simulink model "design_lqr_v1"  (R2019b)
settings: Solver=VariableStepAuto  StartTime=0.0  StopTime=10  RelTol=1e-3
values from neighbouring files (symbols this model uses):
  Ac = [A-B*F B*F;zeros(1*9) A-Ke*C1]    [design_hinfinity.m]    (also in design_lqr_m.m = [A-B*F B*F;zeros(9) A-Ke*C1]; design_v1.m)
  Bc = 1.0e+03*[ ... (first row only)    [design_hinfinity.m]    (also in design_lqr_m.m = [B*G;Zero_tem]; design_v1.m)
  Cc = [ 1     0     0     0     0     0     0     0     0  0     0     0     0     0     0     0     0     0 ... (first row only)    [design_hinfinity.m]    (also in design_lqr_m.m = [C1 zeros(9)]; design_v1.m)
  Rref = [0;0;0]    [design_lqr_m.m]    (also in design_v1.m)
  Vw = [ ... (first row only)    [design_hinfinity.m]    (also in design_lqr_m.m = [E;E]; design_v1.m = [E;E-Ke*[0;0;1;1;0;0;1;0;0]])
  x0 = [0 0 0 0 0 0 0 0 0;0 -0.1 0 0 0 0 0 0 0;0 0 0 0 0 0 0 0 0;0 0 0 0 0 0 0 0 0;0 0 0 0 0 0 0 0 0;0 0 0 0 0 0 0 0 0;0 0 0 0 0 0 0 0 0;0 0 0 0 0 0 0 0 0;0 0 0 0 0 0 0 0  0.1;0 0 0 0 0 0 0 0 0  ;      0 0 0 0 0 0 0 0 0  ;      0 0 0 0 0 0 0 0 0 ;0 0 0 0 0 0 0 0 0   ;      0 0 0 0 0 0 0 0 0    ;     0 0 0 0 0 0 0 0 0;0 0 0 0 0 0 0 0 0;0 0 0 0 0 0 0 0 0;0 0 0 0 0 0 0 0 0]    [design_hinfinity.m]    (also in design_lqr_m.m = [0;-0.1;0;0;0;0;0;0;0.1;0;0;0;0;0;0;0;0;0]; design_v1.m = [0;-0.1;0;0;0;0;0;0;0.1;0;0;0;0;0;0;0;0;0])
libraries: simulink x2
settings Model: Creator=50474  LastModifiedBy=Administrator
settings DataIOCC: ReturnWorkspaceOutputs=off
settings DebuggingCC: ArithmeticOperatorsInVariantConditions=warning
settings SFSimCC: SimUseLocalCustomCode=off  CustomCodeUndefinedFunction=UseInterfaceOnly
settings RTWCC: RTWUseLocalCustomCode=off

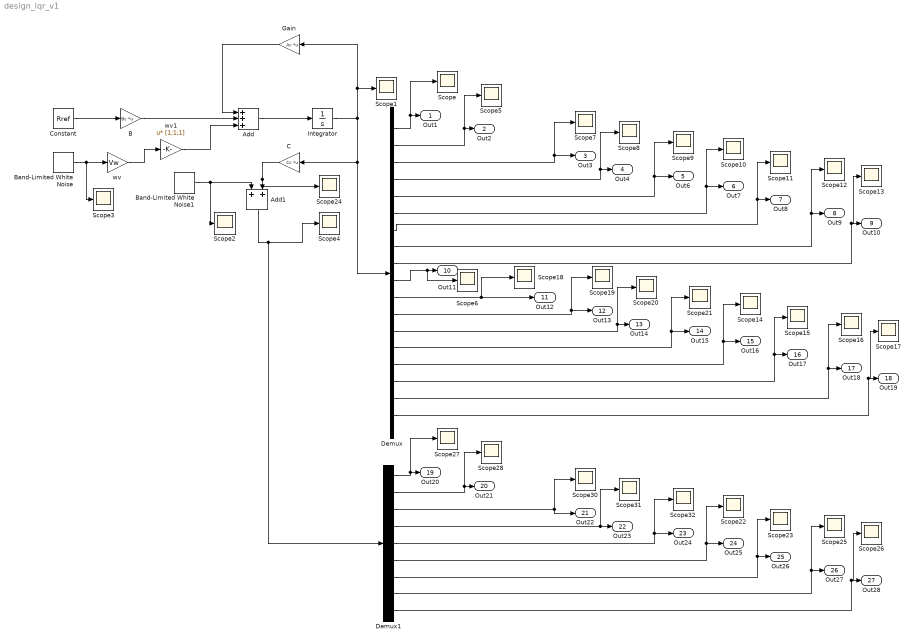
== system design_lqr_v1 ==
  Add : Sum  Inputs=+++
  Add1 : Sum
  B : Gain  Gain=Bc  Multiplication=Matrix(K*u)
  Band-Limited White Noise : simulink/Sources/Band-Limited White Noise  Cov=0.00001  Ts=0.001  seed=[23341]
  Band-Limited White Noise1 : simulink/Sources/Band-Limited White Noise  Cov=[0.00000000001]  Ts=0.001  seed=[23341]
  C : Gain  Gain=Cc  Multiplication=Matrix(K*u)
  Constant : Constant  Value=Rref
  Demux : Demux  Outputs=18
  Demux1 : Demux  Outputs=9
  Gain : Gain  Gain=Ac  Multiplication=Matrix(K*u)
  Integrator : Integrator  InitialCondition=x0
  Scope{,1..28,30..32} (32 alike) : Scope
  wv : Gain  Gain=Vw
  wv1 : Gain  Gain=[1;1;1]  Multiplication=Matrix(u*K)
  Out1 : Outport  VectorParamsAs1DForOutWhenUnconnected=off
  Out2 : Outport  Port=2  VectorParamsAs1DForOutWhenUnconnected=off
  Out3 : Outport  Port=3  VectorParamsAs1DForOutWhenUnconnected=off
  Out4 : Outport  Port=4  VectorParamsAs1DForOutWhenUnconnected=off
  Out6 : Outport  Port=5  VectorParamsAs1DForOutWhenUnconnected=off
  Out7 : Outport  Port=6  VectorParamsAs1DForOutWhenUnconnected=off
  Out8 : Outport  Port=7  VectorParamsAs1DForOutWhenUnconnected=off
  Out9 : Outport  Port=8  VectorParamsAs1DForOutWhenUnconnected=off
  Out10 : Outport  Port=9  VectorParamsAs1DForOutWhenUnconnected=off
  Out11 : Outport  Port=10  VectorParamsAs1DForOutWhenUnconnected=off
  Out12 : Outport  Port=11  VectorParamsAs1DForOutWhenUnconnected=off
  Out13 : Outport  Port=12  VectorParamsAs1DForOutWhenUnconnected=off
  Out14 : Outport  Port=13  VectorParamsAs1DForOutWhenUnconnected=off
  Out15 : Outport  Port=14  VectorParamsAs1DForOutWhenUnconnected=off
  Out16 : Outport  Port=15  VectorParamsAs1DForOutWhenUnconnected=off
  Out17 : Outport  Port=16  VectorParamsAs1DForOutWhenUnconnected=off
  Out18 : Outport  Port=17  VectorParamsAs1DForOutWhenUnconnected=off
  Out19 : Outport  Port=18  VectorParamsAs1DForOutWhenUnconnected=off
  Out20 : Outport  Port=19  VectorParamsAs1DForOutWhenUnconnected=off
  Out21 : Outport  Port=20  VectorParamsAs1DForOutWhenUnconnected=off
  Out22 : Outport  Port=21  VectorParamsAs1DForOutWhenUnconnected=off
  Out23 : Outport  Port=22  VectorParamsAs1DForOutWhenUnconnected=off
  Out24 : Outport  Port=23  VectorParamsAs1DForOutWhenUnconnected=off
  Out25 : Outport  Port=24  VectorParamsAs1DForOutWhenUnconnected=off
  Out26 : Outport  Port=25  VectorParamsAs1DForOutWhenUnconnected=off
  Out27 : Outport  Port=26  VectorParamsAs1DForOutWhenUnconnected=off
  Out28 : Outport  Port=27  VectorParamsAs1DForOutWhenUnconnected=off
  wires:
  Add/1 -> Integrator/1
  Integrator/1 -> Demux/1, C/1, Scope1/1, Gain/1
  Gain/1 -> Add/1
  Constant/1 -> B/1
  B/1 -> Add/2
  Band-Limited White Noise/1 -> Scope3/1, wv/1
  C/1 -> Scope24/1, Add1/2
  Band-Limited White Noise1/1 -> Scope2/1, Add1/1
  Demux/1 -> Scope/1, Out1/1
  Demux/2 -> Out2/1, Scope5/1
  Demux/3 -> Scope7/1, Out3/1
  Demux/4 -> Scope8/1, Out4/1
  Demux/5 -> Scope9/1, Out6/1
  Demux/6 -> Scope10/1, Out7/1
  Demux/7 -> Scope11/1, Out8/1
  Demux/8 -> Scope12/1, Out9/1
  wv/1 -> wv1/1
  wv1/1 -> Add/3
  Demux/9 -> Scope13/1, Out10/1
  Demux/15 -> Scope14/1, Out16/1
  Demux/14 -> Scope21/1, Out15/1
  Demux/12 -> Scope19/1, Out13/1
  Demux/16 -> Scope15/1, Out17/1
  Demux/11 -> Scope18/1, Out12/1
  Demux/17 -> Scope16/1, Out18/1
  Demux/13 -> Scope20/1, Out14/1
  Demux/18 -> Scope17/1, Out19/1
  Demux/10 -> Scope6/1, Out11/1
  Demux1/6 -> Scope22/1, Out25/1
  Demux1/3 -> Out22/1, Scope30/1
  Demux1/2 -> Scope28/1, Out21/1
  Demux1/8 -> Scope25/1, Out27/1
  Demux1/7 -> Scope23/1, Out26/1
  Demux1/1 -> Scope27/1, Out20/1
  Demux1/4 -> Scope31/1, Out23/1
  Add1/1 -> Demux1/1, Scope4/1
  Demux1/5 -> Scope32/1, Out24/1
  Demux1/9 -> Scope26/1, Out28/1
